simulink model "sim_internal_baseline_TB"  (R2025b)
settings: Solver=FixedStepDiscrete  StartTime=0.0  StopTime=10e-3  RelTol=1e-3
PostLoadFcn:
  | hScopeConfig = get_param([gcs '/Receiver/QPSK Rx/Frequency and Time Synchronizer/Symbol Synchronizer/No HDL/QPSK Receiver Eye Diagram'],'ScopeConfiguration');
  | 
  | hScopeConfig.OpenAtSimulationStart = false;
  | hScopeConfig.Visible = false;
  | SamplesPerSymbol = 4;
  | %UpsamplesRx = 1;
  | clear hScopeConfig
InitFcn:
  | commhdlQPSKTxRxModelInit;
  | % Rate bridge: ADRV9002/Jupiter radio runs at 15.36 MHz = 2x the 7.68 MHz
  | % (4 samples/symbol @ Rsym=1.92 MHz) the QPSK Rx requires. The deployed
  | % Receiver must downsample the ADC stream by 2. UpsamplesRx=1 fed the QPSK
  | % Rx 8 sps (2x-upsampled) and broke symbol sync / the loopback bit check.
  | UpsamplesRx = 2;
  | UpsamplesTx = 1;
  | clear simTimingOffset;
StopFcn:
  | if exist('simTimingOffset','var')
  |   disp('Simulation completed');
  |   %QPSKTxRxVerification;
  | end
values from neighbouring files (symbols this model uses):
  Rsym = variant{2}    [BandwidthVariantSimTest.m]    (also in CoarseFreqEstimatorTest.m = CoarseFreqEstimatorTest.Rsym; PreambleDetectorTest.m = 1920000)
undefined symbols (not defined in the file or in its folder): Add, Config, fsym, randsrc, RandStream, Shift
libraries: hdlsllib x149, simulink x40, dspsigops x36, dsphdlfiltering2 x6, dsphdlsigops2 x4, dsphdlmathfun2 x4, commdigbbndpm3 x4, commchan3 x1, commrflib2 x1
(part 2 of 6)

== system sim_internal_baseline_TB/Receiver/QPSK Rx/Frequency and Time Synchronizer ==
  dataIn : Inport
  validIn : Inport  Port=2
  rstCS : Inport  Port=3
  Carrier Synchronizer : Subsystem
      settings: PortSchema="{\"entries\":[{\"content\":{\"sides\":[{\"content\":{\"connectorIds\":[\"In1\",\"In2\",\"In3\"]},\"type\":\"ConnectorPlacement.EquallySpacedRectSide\",\"uuid\":\"ee58e5dc-083a-48cb-b7f3-66ed8a15890f\"},{\"content\":{\"connectorIds\":[\"Out1\",\"Out2\"],\"side\":\"RIGHT\"},\"type\":\"ConnectorPlacement.EquallySpacedRectSide\",\"uuid\":\"6d121164-5065-4840-a82e-fa57a8e9650e\"},{\"content\":{\"connectorIds\":[\"In4\"],\"side\":\"TOP\"},\"type\":\"ConnectorPlacement.EquallySpacedRectSide\",\"uuid\":\"54d2b8e3-f516-4572-94a0-c914196ae8e4\"}]},\"type\":\"ConnectorPlacement.EquallySpacedConnector\",\"uuid\":\"0f2a6472-efd0-42ca-a030-ab436081b5e1\"}],\"packageUris\":[\"http://schema.mathworks.com/mf0/Connector/R2020b\"],\"version\":\"1.0\"}"
  Coarse Frequency Compensator : Subsystem
      settings: PortSchema="{\"entries\":[{\"content\":{\"sides\":[{\"content\":{\"connectorIds\":[\"In1\",\"In2\"]},\"type\":\"ConnectorPlacement.EquallySpacedRectSide\",\"uuid\":\"138aa5bd-62db-47d6-b55f-f529a6004434\"},{\"content\":{\"connectorIds\":[\"Out1\",\"Out2\",\"Out3\"],\"side\":\"RIGHT\"},\"type\":\"ConnectorPlacement.EquallySpacedRectSide\",\"uuid\":\"8e6ccec0-f736-48ab-be6d-feac886e083d\"},{\"content\":{\"connectorIds\":[\"Out4\"],\"side\":\"TOP\"},\"type\":\"ConnectorPlacement.EquallySpacedRectSide\",\"uuid\":\"d4535392-74fa-432a-a39c-b98ba26e8163\"},{\"content\":{\"side\":\"BOTTOM\"},\"type\":\"ConnectorPlacement.EquallySpacedRectSide\",\"uuid\":\"770ac6a2-7a02-4a77-858b-592982deaf6e\"}]},\"type\":\"ConnectorPlacement.EquallySpacedConnector\",\"uuid\":\"a9b944be-f88b-4ab6-a5e1-6824362eb9ca\"}],\"packageUris\":[\"http://schema.mathworks.com/mf0/Connector/R2020b\"],\"version\":\"1.0\"}"
  No HDL : Subsystem
      settings: PortSchema="{\"entries\":[{\"content\":{\"sides\":[{\"content\":{\"connectorIds\":[\"In1\",\"In2\"]},\"type\":\"ConnectorPlacement.EquallySpacedRectSide\",\"uuid\":\"df96a46d-149f-4580-adf6-e5cf26cffa9b\"},{\"content\":{\"connectorIds\":[\"In3\",\"In4\"],\"side\":\"RIGHT\"},\"type\":\"ConnectorPlacement.EquallySpacedRectSide\",\"uuid\":\"1c46d09c-cb37-4618-ac4e-e5ef50df41fb\"},{\"content\":{\"connectorIds\":[],\"side\":\"TOP\"},\"type\":\"ConnectorPlacement.EquallySpacedRectSide\",\"uuid\":\"7fe62300-46d7-4234-a31d-eecffed4f6e6\"},{\"content\":{\"connectorIds\":[],\"side\":\"BOTTOM\"},\"type\":\"ConnectorPlacement.EquallySpacedRectSide\",\"uuid\":\"05ecd563-28f5-4cfd-b718-5032a7458763\"}]},\"type\":\"ConnectorPlacement.EquallySpacedConnector\",\"uuid\":\"4b3d5859-a469-4389-9e5d-e5f07416a9a1\"}],\"packageUris\":[\"http://schema.mathworks.com/mf0/Connector/R2020b\"],\"version\":\"1.0\"}"
  Packet Controller : Subsystem
  Phase Ambiguity Estimation and Correction : Subsystem
  Preamble Detector : Subsystem
  Symbol Synchronizer : Subsystem
  dataOut : Outport
  startOut : Outport  Port=2
  endOut : Outport  Port=3
  validOut : Outport  Port=4
  postSymbolSync : Outport  Port=5
  postCarrierSync : Outport  Port=6
  nSynced : Outport  Port=7
  normCoarseFreqEst : Outport  Port=8
  wires:
  Coarse Frequency Compensator/3(validOut) -> Carrier Synchronizer/3(validIn)
  Coarse Frequency Compensator/1(dataOut) -> Carrier Synchronizer/1(dataIn)
  Phase Ambiguity Estimation and Correction/1(dataOut) -> Packet Controller/1(dataIn)
  Phase Ambiguity Estimation and Correction/3(validOut) -> Packet Controller/3(validIn)
  Symbol Synchronizer/2(validOut) -> No HDL/2(In2), Coarse Frequency Compensator/2(validIn)
  Symbol Synchronizer/1(dataOut) -> postSymbolSync/1, No HDL/1(In1), Coarse Frequency Compensator/1(dataIn)
  Phase Ambiguity Estimation and Correction/2(syncPulseOut) -> Packet Controller/2(syncPulse)
  Preamble Detector/3(validOut) -> Phase Ambiguity Estimation and Correction/3(validIn)
  Preamble Detector/1(dataOut) -> Phase Ambiguity Estimation and Correction/1(dataIn)
  validIn/1 -> Symbol Synchronizer/2(validIn)
  dataIn/1 -> Symbol Synchronizer/1(dataIn)
  Coarse Frequency Compensator/2(rstCS) -> Carrier Synchronizer/2(internalRst)
  Packet Controller/1(dataOut) -> dataOut/1
  Packet Controller/2(startOut) -> startOut/1
  Packet Controller/3(endOut) -> endOut/1
  Packet Controller/4(validOut) -> validOut/1
  Preamble Detector/2(syncPulse) -> nSynced/1, Phase Ambiguity Estimation and Correction/2(syncPulseIn)
  Carrier Synchronizer/1(dataOut) -> postCarrierSync/1, No HDL/3(In3), Preamble Detector/1(dataIn)
  Carrier Synchronizer/2(validOut) -> No HDL/4(In4), Preamble Detector/2(validIn)
  Coarse Frequency Compensator/4(normalizedFreqEst) -> normCoarseFreqEst/1
  rstCS/1 -> Carrier Synchronizer/4(manualRst)

== system sim_internal_baseline_TB/Receiver/QPSK Rx/HDL Data Descrambler ==
  note: HDL Data Scrambler
      | Polynomial: x^7+x^4+1
      | Initial state: [1 0 1 1 1 0 1]
  dataIn : Inport
  startIn : Inport  Port=2
  endIn : Inport  Port=3
  validIn : Inport  Port=4
  BIT_XOR : Logic  Operator=XOR  IconShape=distinctive  AllPortsSameDT=off  OutDataTypeStr=boolean
  BIT_XOR2 : Logic  Operator=XOR  IconShape=distinctive  AllPortsSameDT=off  OutDataTypeStr=boolean
  Delay{,1..7} (8 alike) : Delay  DelayLength=1
  EnableScrambling : Constant  Value=true  SampleTime=-1
  Logical Operator : Logic  IconShape=distinctive  AllPortsSameDT=off  OutDataTypeStr=boolean
  Switch : Switch  Criteria=u2 > Threshold  SaturateOnIntegerOverflow=off  InputSameDT=off
  Unit Delay Enabled Resettable Synchronous{,2..3,5,7} (5 alike) : hdlsllib/Discrete/Unit Delay Enabled Resettable Synchronous  InitialCondition=1  SampleTime=-1
  Unit Delay Enabled Resettable Synchronous1 : hdlsllib/Discrete/Unit Delay Enabled Resettable Synchronous  InitialCondition=0  SampleTime=-1
  Unit Delay Enabled Resettable Synchronous4 : hdlsllib/Discrete/Unit Delay Enabled Resettable Synchronous  InitialCondition=0  SampleTime=-1
  Unit Delay Enabled Resettable Synchronous6 : hdlsllib/Discrete/Unit Delay Enabled Resettable Synchronous  InitialCondition=0.0  SampleTime=-1
  dataOut : Outport  InitialOutput=0
  startOut : Outport  Port=2  InitialOutput=0
  endOut : Outport  Port=3  InitialOutput=0
  validOut : Outport  Port=4  InitialOutput=0
  wires:
  Delay4/1 -> validOut/1
  Delay3/1 -> dataOut/1
  endIn/1 -> Delay2/1, Unit Delay Enabled Resettable Synchronous4/3
  Logical Operator/1 -> BIT_XOR2/2
  Unit Delay Enabled Resettable Synchronous4/1 -> Logical Operator/1
  Delay1/1 -> Unit Delay Enabled Resettable Synchronous6/2, Unit Delay Enabled Resettable Synchronous2/2, Unit Delay Enabled Resettable Synchronous1/2, Unit Delay Enabled Resettable Synchronous/2, Delay4/1, Unit Delay Enabled Resettable Synchronous3/2, Unit Delay Enabled Resettable Synchronous5/2, Unit Delay Enabled Resettable Synchronous7/2
  Delay/1 -> Switch/3, BIT_XOR2/1
  startIn/1 -> Delay5/1, Unit Delay Enabled Resettable Synchronous4/1, Unit Delay Enabled Resettable Synchronous4/2, Unit Delay Enabled Resettable Synchronous6/3, Unit Delay Enabled Resettable Synchronous5/3, Unit Delay Enabled Resettable Synchronous1/3, Unit Delay Enabled Resettable Synchronous/3, Unit Delay Enabled Resettable Synchronous2/3, Unit Delay Enabled Resettable Synchronous3/3, Unit Delay Enabled Resettable Synchronous7/3
  dataIn/1 -> Delay/1
  validIn/1 -> Delay1/1
  BIT_XOR/1 -> Unit Delay Enabled Resettable Synchronous/1, Logical Operator/2
  Unit Delay Enabled Resettable Synchronous1/1 -> Unit Delay Enabled Resettable Synchronous2/1
  Unit Delay Enabled Resettable Synchronous2/1 -> Unit Delay Enabled Resettable Synchronous3/1
  Unit Delay Enabled Resettable Synchronous/1 -> Unit Delay Enabled Resettable Synchronous1/1
  Unit Delay Enabled Resettable Synchronous3/1 -> BIT_XOR/2, Unit Delay Enabled Resettable Synchronous5/1
  Unit Delay Enabled Resettable Synchronous5/1 -> Unit Delay Enabled Resettable Synchronous6/1
  Unit Delay Enabled Resettable Synchronous6/1 -> Unit Delay Enabled Resettable Synchronous7/1
  Unit Delay Enabled Resettable Synchronous7/1 -> BIT_XOR/1
  Delay2/1 -> Delay6/1
  Delay5/1 -> Delay7/1
  Delay6/1 -> endOut/1
  Delay7/1 -> startOut/1
  EnableScrambling/1 -> Switch/2
  BIT_XOR2/1 -> Switch/1
  Switch/1 -> Delay3/1

== system sim_internal_baseline_TB/Receiver/QPSK Rx/QPSK Demodulator ==
  dataIn : Inport
  startIn : Inport  Port=2
  endIn : Inport  Port=3
  validIn : Inport  Port=4
  Delay{,1..13} (14 alike) : Delay  DelayLength=1
  QPSK Demodulator Baseband : commdigbbndpm3/QPSK Demodulator Baseband  OutType=Bit  DecType=Hard decision  VarSource=Dialog  Variance=1  Dec=Gray  Ph=pi/4  outDtype1=boolean  outDtype2=Inherit via internal rule  derotateFactorWordLen=16  derotateFactorDataTypeStr=Inherit: Same word length as input  derotateFactorLastDataTypeStr=Inherit: Same word length as input
  Serializer : Subsystem
  Signal Specification : SignalSpecification  Dimensions=1
  dataOut : Outport
  startOut : Outport  Port=2
  endOut : Outport  Port=3
  validOut : Outport  Port=4
  wires:
  Delay/1 -> QPSK Demodulator Baseband/1
  Delay1/1 -> Delay5/1
  Delay6/1 -> Delay4/1
  Delay7/1 -> Delay13/1
  Delay2/1 -> Delay6/1
  Delay3/1 -> Delay7/1
  Signal Specification/1 -> Delay/1
  QPSK Demodulator Baseband/1 -> Delay12/1
  Delay8/1 -> dataOut/1
  Delay9/1 -> validOut/1
  Delay10/1 -> startOut/1
  Delay11/1 -> endOut/1
  Delay5/1 -> Serializer/2(In2)
  Delay12/1 -> Serializer/1(u)
  Delay4/1 -> Delay10/1
  Delay13/1 -> Delay11/1
  Serializer/1(Out1) -> Delay8/1
  Serializer/2(Out2) -> Delay9/1
  dataIn/1 -> Signal Specification/1
  validIn/1 -> Delay1/1
  startIn/1 -> Delay2/1
  endIn/1 -> Delay3/1

== system sim_internal_baseline_TB/Transmitter/Input Data/Message Generator ==
  reset : Inport
  enable : Inport  Port=2
  MATLAB Function : MATLAB Function  TreatAsAtomicUnit=on
  out : Outport
  stop : Outport  Port=2
  start : Outport  Port=3
  valid : Outport  Port=4
  count : Outport  Port=5
  msg_count_out : Outport  Port=6
  wires:
  MATLAB Function/3(stop) -> stop/1
  MATLAB Function/1(out) -> out/1
  reset/1 -> MATLAB Function/2(reset)
  MATLAB Function/2(start) -> start/1
  enable/1 -> MATLAB Function/1(enable)
  MATLAB Function/4(valid) -> valid/1
  MATLAB Function/5(count_out) -> count/1
  MATLAB Function/6(msg_count_out) -> msg_count_out/1

== system sim_internal_baseline_TB/Transmitter/QPSK Tx/Bit Packetizer ==
  dataIn : Inport
  validIn : Inport  Port=2
  Compare To Constant : hdlsllib/Logic and Bit Operations/Compare To Constant  relop===  const=length(Preamble)  OutDataTypeStr=boolean
  Compare To Constant1 : hdlsllib/Logic and Bit Operations/Compare To Constant  relop===  const=bitsPerPacket - 1  OutDataTypeStr=boolean
  Compare To Constant2 : hdlsllib/Logic and Bit Operations/Compare To Constant  relop=>=  const=length(Preamble)  OutDataTypeStr=boolean
  Data Bits FIFO : Subsystem
  Data Type Conversion : DataTypeConversion  OutDataTypeStr=boolean  SaturateOnIntegerOverflow=off  RndMeth=Floor
  HDL Counter : hdlsllib/Sources/HDL Counter  CountType=Count limited  CountInit=0  CountStep=1  CountMax=1  CountFromType=Initial value  CountFrom=0  CountResetPort=off  CountLoadPort=off  CountEnbPort=on  CountDirPort=off  CountHitOutputPort=off  CountDataType=Unsigned  CountWordLen=1  CountFracLen=0  CountSampTime=1
  Logical Operator : Logic  AllPortsSameDT=off  OutDataTypeStr=boolean
  Logical Operator1 : Logic  AllPortsSameDT=off  OutDataTypeStr=boolean
  Logical Operator2 : Logic  Operator=NOT  AllPortsSameDT=off  OutDataTypeStr=boolean
  Preamble Bits Generator : Subsystem
  Switch : Switch  Criteria=u2 ~= 0  SaturateOnIntegerOverflow=off  InputSameDT=off
  bitsOut : Outport
  dataStart : Outport  Port=2
  dataEnd : Outport  Port=3
  bitsValid : Outport  Port=4
  dataReady : Outport  Port=5
  wires:
  dataIn/1 -> Data Bits FIFO/1(data)
  validIn/1 -> Data Bits FIFO/2(push)
  Compare To Constant/1 -> Logical Operator/1
  Compare To Constant1/1 -> Logical Operator1/2
  Logical Operator/1 -> dataStart/1
  Logical Operator1/1 -> dataEnd/1
  Data Bits FIFO/5(fullRAM) -> Logical Operator2/1
  Logical Operator2/1 -> HDL Counter/1
  Data Bits FIFO/1(dataOut) -> Switch/1
  Data Bits FIFO/3(sampleCount) -> Preamble Bits Generator/2(sampleCount), Compare To Constant/1, Compare To Constant1/1, Compare To Constant2/1
  Data Bits FIFO/4(sampleCountValid) -> bitsValid/1, Logical Operator/2, Logical Operator1/1, Preamble Bits Generator/3(sampleCountValid)
  Data Bits FIFO/2(activeFrame) -> Preamble Bits Generator/1(activeFrame)
  Preamble Bits Generator/1(preambleBits) -> Switch/3
  Compare To Constant2/1 -> Switch/2
  Switch/1 -> bitsOut/1
  HDL Counter/1 -> Data Type Conversion/1
  Data Type Conversion/1 -> dataReady/1

== system sim_internal_baseline_TB/Transmitter/QPSK Tx/HDL Data Scrambler ==
  note: HDL Data Scrambler
      | Polynomial: x^7+x^4+1
      | Initial state: [1 0 1 1 1 0 1]
  dataIn : Inport
  startIn : Inport  Port=2
  endIn : Inport  Port=3
  validIn : Inport  Port=4
  BIT_XOR : Logic  Operator=XOR  IconShape=distinctive  AllPortsSameDT=off  OutDataTypeStr=boolean
  BIT_XOR2 : Logic  Operator=XOR  IconShape=distinctive  AllPortsSameDT=off  OutDataTypeStr=boolean
  Delay{,1,3..4} (4 alike) : Delay  DelayLength=1
  EnableScrambling : Constant  Value=true  SampleTime=-1
  Logical Operator : Logic  IconShape=distinctive  AllPortsSameDT=off  OutDataTypeStr=boolean
  Switch : Switch  Criteria=u2 > Threshold  SaturateOnIntegerOverflow=off  InputSameDT=off
  Unit Delay Enabled Resettable Synchronous{,2..3,5,7} (5 alike) : hdlsllib/Discrete/Unit Delay Enabled Resettable Synchronous  InitialCondition=1  SampleTime=-1
  Unit Delay Enabled Resettable Synchronous1 : hdlsllib/Discrete/Unit Delay Enabled Resettable Synchronous  InitialCondition=0  SampleTime=-1
  Unit Delay Enabled Resettable Synchronous4 : hdlsllib/Discrete/Unit Delay Enabled Resettable Synchronous  InitialCondition=0  SampleTime=-1
  Unit Delay Enabled Resettable Synchronous6 : hdlsllib/Discrete/Unit Delay Enabled Resettable Synchronous  InitialCondition=0.0  SampleTime=-1
  dataOut : Outport  InitialOutput=0
  validOut : Outport  Port=2  InitialOutput=0
  wires:
  Delay4/1 -> validOut/1
  Delay3/1 -> dataOut/1
  endIn/1 -> Unit Delay Enabled Resettable Synchronous4/3
  Logical Operator/1 -> BIT_XOR2/2
  Unit Delay Enabled Resettable Synchronous4/1 -> Logical Operator/1
  Delay1/1 -> Unit Delay Enabled Resettable Synchronous6/2, Unit Delay Enabled Resettable Synchronous2/2, Unit Delay Enabled Resettable Synchronous1/2, Unit Delay Enabled Resettable Synchronous/2, Delay4/1, Unit Delay Enabled Resettable Synchronous3/2, Unit Delay Enabled Resettable Synchronous5/2, Unit Delay Enabled Resettable Synchronous7/2
  Delay/1 -> Switch/3, BIT_XOR2/1
  startIn/1 -> Unit Delay Enabled Resettable Synchronous4/1, Unit Delay Enabled Resettable Synchronous4/2, Unit Delay Enabled Resettable Synchronous6/3, Unit Delay Enabled Resettable Synchronous5/3, Unit Delay Enabled Resettable Synchronous1/3, Unit Delay Enabled Resettable Synchronous/3, Unit Delay Enabled Resettable Synchronous2/3, Unit Delay Enabled Resettable Synchronous3/3, Unit Delay Enabled Resettable Synchronous7/3
  dataIn/1 -> Delay/1
  validIn/1 -> Delay1/1
  BIT_XOR/1 -> Unit Delay Enabled Resettable Synchronous/1, Logical Operator/2
  Unit Delay Enabled Resettable Synchronous1/1 -> Unit Delay Enabled Resettable Synchronous2/1
  Unit Delay Enabled Resettable Synchronous2/1 -> Unit Delay Enabled Resettable Synchronous3/1
  Unit Delay Enabled Resettable Synchronous/1 -> Unit Delay Enabled Resettable Synchronous1/1
  Unit Delay Enabled Resettable Synchronous3/1 -> BIT_XOR/2, Unit Delay Enabled Resettable Synchronous5/1
  Unit Delay Enabled Resettable Synchronous5/1 -> Unit Delay Enabled Resettable Synchronous6/1
  Unit Delay Enabled Resettable Synchronous6/1 -> Unit Delay Enabled Resettable Synchronous7/1
  Unit Delay Enabled Resettable Synchronous7/1 -> BIT_XOR/1
  Switch/1 -> Delay3/1
  EnableScrambling/1 -> Switch/2
  BIT_XOR2/1 -> Switch/1

== system sim_internal_baseline_TB/Transmitter/QPSK Tx/QPSK Modulator ==
  dataIn : Inport
  validIn : Inport  Port=2
  Compare To Constant : simulink/Logic and Bit Operations/Compare To Constant  relop===  const=0  OutDataTypeStr=boolean
  Compare To Constant1 : simulink/Logic and Bit Operations/Compare To Constant  relop===  const=1  OutDataTypeStr=boolean
  Delay{,1..5,11..12} (8 alike) : Delay  DelayLength=1
  HDL Counter : hdlsllib/Sources/HDL Counter  CountType=Count limited  CountInit=0  CountStep=1  CountMax=1  CountFromType=Initial value  CountFrom=0  CountResetPort=off  CountLoadPort=off  CountEnbPort=on  CountDirPort=off  CountHitOutputPort=off  CountDataType=Unsigned  CountWordLen=1  CountFracLen=0  CountSampTime=1
  Logical Operator : Logic  IconShape=distinctive  AllPortsSameDT=off  OutDataTypeStr=boolean
  Logical Operator1 : Logic  IconShape=distinctive  AllPortsSameDT=off  OutDataTypeStr=boolean
  Mux : Mux  Inputs=2
  Null : Constant  Value=complex(0,0)  OutDataTypeStr=fixdt(1,16,15)  SampleTime=1/(Rsym*4)
  QPSK Modulator Baseband : commdigbbndpm3/QPSK Modulator Baseband  InType=Bit  Enc=Gray  Ph=pi/4  outDtype=Fixed-point  outWordLen=16  outUDDataType=sfix(16)  outFracLenMode=User-defined  outFracLen=15  outDataTypeStr=fixdt(1,16,15)  outLastDataTypeStr=fixdt(1,16,15)
  Switch3 : Switch  Threshold=1  SaturateOnIntegerOverflow=off  InputSameDT=off
  Unit Delay Enabled Synchronous : hdlsllib/Discrete/Unit Delay Enabled Synchronous  InitialCondition=0.0  SampleTime=-1
  dataOut : Outport
  validOut : Outport  Port=2
  wires:
  dataIn/1 -> Delay/1
  validIn/1 -> Delay1/1
  HDL Counter/1 -> Compare To Constant/1, Compare To Constant1/1
  QPSK Modulator Baseband/1 -> Delay11/1
  Logical Operator1/1 -> Delay5/1
  Switch3/1 -> Delay2/1
  Null/1 -> Switch3/3
  Delay/1 -> Mux/2, Unit Delay Enabled Synchronous/1
  Delay2/1 -> dataOut/1
  Delay3/1 -> validOut/1
  Delay1/1 -> Logical Operator1/2, Logical Operator/1, HDL Counter/1
  Compare To Constant/1 -> Logical Operator/2
  Compare To Constant1/1 -> Logical Operator1/1
  Delay11/1 -> Switch3/1
  Delay12/1 -> Switch3/2, Delay3/1
  Logical Operator/1 -> Unit Delay Enabled Synchronous/2
  Unit Delay Enabled Synchronous/1 -> Mux/1
  Mux/1 -> Delay4/1
  Delay4/1 -> QPSK Modulator Baseband/1
  Delay5/1 -> Delay12/1

== system sim_internal_baseline_TB/Transmitter/QPSK Tx/RRC Transmit Filter ==
  dataIn : Inport
  validIn : Inport  Port=2
  Data Type Conversion : DataTypeConversion  OutDataTypeStr=fixdt(1,17,16)  SaturateOnIntegerOverflow=off  RndMeth=Floor
  Data Type Conversion1 : DataTypeConversion  OutDataTypeStr=fixdt(1,16,14)  SaturateOnIntegerOverflow=off  RndMeth=Floor
  Delay1 : Delay  DelayLength=1
  Delay2 : Delay  DelayLength=1
  Delay3 : Delay  DelayLength=1
  RRC Filter : dsphdlfiltering2/Discrete FIR Filter  NumeratorSource=Property  Numerator=RRCCoef  NumeratorPrototype=[]  FilterStructure=Direct form systolic  SerializationOption=Minimum number of cycles between valid input samples  NumCycles=2  NumberOfMultipliers=2  SimulateUsing=Code generation  roundingMode=Floor  overflowMode=off  CoefficientsDataTypeStr=Inherit: Same word length as input  OutputDataTypeStr=Inherit: Same word length as input  ResetInputPort=off  HDLGlobalReset=off  CoeffMultiplier=Multiplier  UseMultForPow2Coeff=on  FrameInputSymmOptim=off
  Unit Delay Enabled Synchronous1 : hdlsllib/Discrete/Unit Delay Enabled Synchronous  InitialCondition=0  SampleTime=-1
  dataOut : Outport
  validOut : Outport  Port=2
  wires:
  dataIn/1 -> Data Type Conversion/1
  RRC Filter/1 -> Data Type Conversion1/1
  RRC Filter/2 -> Delay2/1
  Delay1/1 -> dataOut/1
  Delay2/1 -> validOut/1
  Data Type Conversion/1 -> Delay3/1
  Unit Delay Enabled Synchronous1/1 -> RRC Filter/2
  Data Type Conversion1/1 -> Delay1/1
  validIn/1 -> Unit Delay Enabled Synchronous1/2, Unit Delay Enabled Synchronous1/1
  Delay3/1 -> RRC Filter/1

== system sim_internal_baseline_TB/TxRxComposite/Receiver/Capture Data Bits ==
  dataOut : Inport
  dataSrt : Inport  Port=2
  dataEnd : Inport  Port=3
  valid : Inport  Port=4
  Display : Display
  Display1 : Display
  Display2 : Display
  MATLAB Function : MATLAB Function  TreatAsAtomicUnit=on
  count_out : Outport
  packets_out : Outport  Port=2
  bit_errors_out : Outport  Port=3
  wires:
  MATLAB Function/3(bit_errors_out) -> Display2/1, bit_errors_out/1
  MATLAB Function/2(packets_out) -> Display1/1, packets_out/1
  MATLAB Function/1(count_out) -> Display/1, count_out/1
  valid/1 -> MATLAB Function/1(valid)
  dataEnd/1 -> MATLAB Function/4(stop)
  dataSrt/1 -> MATLAB Function/3(start)
  dataOut/1 -> MATLAB Function/2(datain)

== system sim_internal_baseline_TB/TxRxComposite/Receiver/QPSK Rx ==
  dataIn : Inport  OutDataTypeStr=fixdt(1,16,14)  PortDimensions=1  SampleTime=1/(Rsym*SamplesPerSymbol)
      settings: SignalType=complex
  validIn : Inport  Port=2  OutDataTypeStr=boolean  PortDimensions=1  SampleTime=1/(Rsym*SamplesPerSymbol)
  rstCS : Inport  Port=3  OutDataTypeStr=boolean  PortDimensions=1
      settings: SignalType=complex
  debugMuxCtrl : Inport  Port=4  OutDataTypeStr=uint32  PortDimensions=1  SampleTime=1/(Rsym*SamplesPerSymbol)
  Automatic Gain Control : Subsystem  mask{Ref=AGCReference, LFG=AGCLoopGain}
      mask prompts: Ref "Error Detector Reference:"; LFG "Loop Filter Gain"
  Bus Creator : BusCreator  Inputs=4
  Bus Creator1 : BusCreator  Inputs=3
  Complex to Real-Imag : ComplexToRealImag
  Constant : Constant  Value=true  SampleTime=1/(Rsym*4)
  Data Type Conversion : DataTypeConversion  OutDataTypeStr=int16  ConvertRealWorld=Stored Integer (SI)  SaturateOnIntegerOverflow=off  RndMeth=Floor
  Delay{,1..8} (9 alike) : Delay  DelayLength=1
  Frequency and Time Synchronizer : Subsystem
      settings: PortSchema="{\"entries\":[{\"content\":{\"sides\":[{\"content\":{\"connectorIds\":[\"In1\",\"In2\"]},\"type\":\"ConnectorPlacement.EquallySpacedRectSide\",\"uuid\":\"8bc6a452-5111-4806-8ca9-335cb622aea6\"},{\"content\":{\"connectorIds\":[\"Out1\",\"Out2\",\"Out3\",\"Out4\"],\"side\":\"RIGHT\"},\"type\":\"ConnectorPlacement.EquallySpacedRectSide\",\"uuid\":\"b0f43c98-f5c0-4f62-94ae-d69789942eef\"},{\"content\":{\"connectorIds\":[\"In3\",\"Out7\",\"Out8\"],\"side\":\"TOP\"},\"type\":\"ConnectorPlacement.EquallySpacedRectSide\",\"uuid\":\"427ff3b3-b896-4008-9584-d311480df763\"},{\"content\":{\"connectorIds\":[\"Out5\",\"Out6\"],\"side\":\"BOTTOM\"},\"type\":\"ConnectorPlacement.EquallySpacedRectSide\",\"uuid\":\"f704cb90-80a1-4198-8b72-e70182b45e73\"},{\"content\":{\"side\":\"HIDDEN\"},\"type\":\"ConnectorPlacement.EquallySpacedRectSide\",\"uuid\":\"f6309498-1e43-486f-b6b5-2c6570711f8e\"}]},\"type\":\"ConnectorPlacement.EquallySpacedConnector\",\"uuid\":\"f0ce492e-c9e1-4b35-98ef-84d77b696cfe\"}],\"packageUris\":[\"http://schema.mathworks.com/mf0/Connector/R2020b\"],\"version\":\"1.0\"}"
  HDL Data Descrambler : Subsystem
  Index Vector : MultiPortSwitch  DataPortOrder=Zero-based contiguous  Inputs=4  DiagnosticForDefault=None  zeroidx=on  SaturateOnIntegerOverflow=off  InputSameDT=off
  QPSK Demodulator : Subsystem
  RRC Receive Filter : dsphdlfiltering2/Discrete FIR Filter  NumeratorSource=Property  Numerator=RRCCoef  NumeratorPrototype=[]  FilterStructure=Direct form systolic  SerializationOption=Minimum number of cycles between valid input samples  NumCycles=2  NumberOfMultipliers=2  SimulateUsing=Code generation  roundingMode=Floor  overflowMode=off  CoefficientsDataTypeStr=Inherit: Same word length as input  OutputDataTypeStr=Inherit: Same word length as input  ResetInputPort=off  HDLGlobalReset=off  CoeffMultiplier=Multiplier  UseMultForPow2Coeff=on  FrameInputSymmOptim=off
  dataOut : Outport
  ctrlOut : Outport  Port=2
  rxDiagBus : Outport  Port=3
  debugIOut : Outport  Port=4
  debugQOut : Outport  Port=5
  debugValid : Outport  Port=6
  wires:
  Constant/1 -> Delay8/1
  Delay8/1 -> Delay7/1
  Delay7/1 -> debugValid/1
  Delay6/1 -> Complex to Real-Imag/1
  Index Vector/1 -> Delay5/1
  Delay5/1 -> Data Type Conversion/1
  Delay4/1 -> Index Vector/5
  Delay3/1 -> Index Vector/4
  Delay2/1 -> Index Vector/3
  Delay1/1 -> Index Vector/2
  Data Type Conversion/1 -> Delay6/1
  Complex to Real-Imag/1 -> debugIOut/1
  Complex to Real-Imag/2 -> debugQOut/1
  debugMuxCtrl/1 -> Index Vector/1
  Frequency and Time Synchronizer/6(postCarrierSync) -> Delay3/1
  Frequency and Time Synchronizer/5(postSymbolSync) -> Delay2/1
  Delay/1 -> rxDiagBus/1
  QPSK Demodulator/4(validOut) -> HDL Data Descrambler/4(validIn)
  Frequency and Time Synchronizer/4(validOut) -> Bus Creator/4, QPSK Demodulator/4(validIn)  "QPSKConstellationValid"
  Frequency and Time Synchronizer/2(startOut) -> QPSK Demodulator/2(startIn)
  QPSK Demodulator/2(startOut) -> HDL Data Descrambler/2(startIn)
  HDL Data Descrambler/4(validOut) -> Bus Creator1/3  "validOut"
  HDL Data Descrambler/1(dataOut) -> dataOut/1
  dataIn/1 -> Automatic Gain Control/1(dataIn)
  Frequency and Time Synchronizer/1(dataOut) -> Bus Creator/3, QPSK Demodulator/1(dataIn), Delay4/1  "QPSKConstellationPoints"
  Automatic Gain Control/1(dataOut) -> RRC Receive Filter/1, Delay1/1
  Bus Creator/1 -> Delay/1
  Frequency and Time Synchronizer/7(nSynced) -> Bus Creator/1  "nSynced"
  RRC Receive Filter/2 -> Frequency and Time Synchronizer/2(validIn)
  Frequency and Time Synchronizer/3(endOut) -> QPSK Demodulator/3(endIn)
  HDL Data Descrambler/2(startOut) -> Bus Creator1/1  "startOut"
  Bus Creator1/1 -> ctrlOut/1
  Frequency and Time Synchronizer/8(normCoarseFreqEst) -> Bus Creator/2  "normCoarseFreqEst"
  QPSK Demodulator/3(endOut) -> HDL Data Descrambler/3(endIn)
  HDL Data Descrambler/3(endOut) -> Bus Creator1/2  "endOut"
  RRC Receive Filter/1 -> Frequency and Time Synchronizer/1(dataIn)
  Automatic Gain Control/2(validOut) -> RRC Receive Filter/2
  validIn/1 -> Automatic Gain Control/2(validIn)
  QPSK Demodulator/1(dataOut) -> HDL Data Descrambler/1(dataIn)
  rstCS/1 -> Frequency and Time Synchronizer/3(rstCS)

== system sim_internal_baseline_TB/TxRxComposite/Transmitter/Input Data ==
  enb : Inport
  reset : Inport  Port=2
  Cast To Boolean : DataTypeConversion  OutDataTypeStr=boolean  SaturateOnIntegerOverflow=off  RndMeth=Floor
  Delay : Delay  DelayLength=1
  Display : Display
  Message Generator : Subsystem
  Terminator : Terminator
  Terminator1 : Terminator
  txData : Outport
  txValid : Outport  Port=2
  msg_count_out : Outport  Port=3
  wires:
  Message Generator/6(msg_count_out) -> msg_count_out/1
  Message Generator/3(start) -> Terminator1/1
  reset/1 -> Terminator/1
  Cast To Boolean/1 -> Message Generator/1(reset)
  Delay/1 -> Cast To Boolean/1
  Message Generator/2(stop) -> Delay/1
  Message Generator/5(count) -> Display/1
  enb/1 -> Message Generator/2(enable)
  Message Generator/1(out) -> txData/1
  Message Generator/4(valid) -> txValid/1

== system sim_internal_baseline_TB/TxRxComposite/Transmitter/QPSK Tx ==
  dataIn : Inport  OutDataTypeStr=boolean  PortDimensions=1
  validIn : Inport  Port=2  OutDataTypeStr=boolean  PortDimensions=1
  Bit Packetizer : Subsystem
  Bus Creator : BusCreator  Inputs=2
  HDL Data Scrambler : Subsystem
  QPSK Modulator : Subsystem
  RRC Transmit Filter : Subsystem
  dataReady : Outport
  dataOut : Outport  Port=2
  txDiagBus : Outport  Port=3
  validOut : Outport  Port=4
  wires:
  Bit Packetizer/4(bitsValid) -> HDL Data Scrambler/4(validIn)
  Bus Creator/1 -> txDiagBus/1
  Bit Packetizer/5(dataReady) -> dataReady/1
  Bit Packetizer/2(dataStart) -> HDL Data Scrambler/2(startIn)
  QPSK Modulator/1(dataOut) -> RRC Transmit Filter/1(dataIn), Bus Creator/1  "QPSKConstellationPoints"
  RRC Transmit Filter/1(dataOut) -> dataOut/1
  HDL Data Scrambler/2(validOut) -> QPSK Modulator/2(validIn)
  Bit Packetizer/3(dataEnd) -> HDL Data Scrambler/3(endIn)
  dataIn/1 -> Bit Packetizer/1(dataIn)
  QPSK Modulator/2(validOut) -> RRC Transmit Filter/2(validIn), Bus Creator/2  "QPSKConstellationValid"
  Bit Packetizer/1(bitsOut) -> HDL Data Scrambler/1(dataIn)
  HDL Data Scrambler/1(dataOut) -> QPSK Modulator/1(dataIn)
  RRC Transmit Filter/2(validOut) -> validOut/1
  validIn/1 -> Bit Packetizer/2(validIn)

== system sim_internal_baseline_TB/Receiver/QPSK Rx/Automatic Gain Control/Error Detector ==
  dataIn : Inport
  Add1 : Sum  Inputs=+-
  Conj : Math  Operator=conj
  Data Type Duplicate : DataTypeDuplicate
  Delay{,1..3} (4 alike) : Delay
  Product : Product
  Ref : Constant  Value=Ref  OutDataTypeStr=Inherit: Inherit via back propagation  SampleTime=-1
  err : Outport
  wires:
  Delay3/1 -> err/1
  Delay2/1 -> Add1/2
  Delay1/1 -> Product/1
  Delay/1 -> Product/2
  Ref/1 -> Data Type Duplicate/1, Add1/1
  Conj/1 -> Delay/1
  Product/1 -> Delay2/1
  dataIn/1 -> Conj/1, Data Type Duplicate/2, Delay1/1
  Add1/1 -> Delay3/1

== system sim_internal_baseline_TB/Receiver/QPSK Rx/Automatic Gain Control/Loop Filter ==
  note: Fixed point precision loss warnings
      | are supressed in Mask Init Callback
  err : Inport
  Add : Sum  Inputs=|++  OutDataTypeStr=Inherit: Same as first input
  Delay1 : Delay  DelayLength=1
  Delay2 : Delay
  Delay3 : Delay
  Gain1 : Gain  Gain=LFG  OutDataTypeStr=Inherit: Same as input
      mask init:
      | Simulink.suppressDiagnostic(gcb, 'SimulinkFixedPoint:util:fxpParameterPrecisionLoss');
  gain : Outport
  wires:
  Delay3/1 -> Gain1/1
  Delay2/1 -> Add/1
  Gain1/1 -> Delay2/1
  Add/1 -> Delay1/1
  Delay1/1 -> Add/2, gain/1
  err/1 -> Delay3/1

== system sim_internal_baseline_TB/Receiver/QPSK Rx/Frequency and Time Synchronizer/Carrier Synchronizer ==
  dataIn : Inport
  internalRst : Inport  Port=2
  validIn : Inport  Port=3
  manualRst : Inport  Port=4
  Data Type Conversion2 : DataTypeConversion  OutDataTypeStr=fixdt(1,16,14)  SaturateOnIntegerOverflow=off  RndMeth=Floor
  Delay{,2,5,7,11} (5 alike) : Delay  DelayLength=1
  Delay{1,10,14..15} (4 alike) : Delay  DelayLength=6
  Delay{3..4,6,8..9,12..13} (7 alike) : Delay
  Direct Digital Synthesis : Subsystem
  Logical Operator : Logic  AllPortsSameDT=off  OutDataTypeStr=boolean
  Loop Filter : Subsystem
  Math Function : Math  Operator=conj  SignedPower=on  RndMeth=Zero
  Phase Error Detector : Subsystem
  Product : Product
  dataOut : Outport
  validOut : Outport  Port=2
  wires:
  Delay/1 -> Phase Error Detector/1(dataIn)
  Math Function/1 -> Delay3/1
  Data Type Conversion2/1 -> Delay5/1, Delay/1
  Delay3/1 -> Product/2
  Product/1 -> Delay6/1
  Delay8/1 -> Delay2/1, Delay7/1
  Delay9/1 -> Delay8/1
  Delay4/1 -> Product/1
  Delay6/1 -> Data Type Conversion2/1
  Direct Digital Synthesis/1(expOut) -> Math Function/1
  Loop Filter/1(v) -> Direct Digital Synthesis/3(phaseInc)
  Phase Error Detector/1(PhaseError) -> Loop Filter/1(e)
  Delay2/1 -> Delay1/1
  Delay1/1 -> Loop Filter/2(validIn)
  Delay10/1 -> Delay4/1
  Delay11/1 -> Delay15/1
  Delay12/1 -> Delay11/1
  Delay13/1 -> Delay12/1
  Loop Filter/2(valid) -> Direct Digital Synthesis/2(validIn)
  Delay5/1 -> dataOut/1
  Delay7/1 -> validOut/1
  dataIn/1 -> Delay10/1
  internalRst/1 -> Delay13/1
  validIn/1 -> Delay14/1
  Delay14/1 -> Delay9/1
  manualRst/1 -> Logical Operator/1, Loop Filter/4(externalRst)
  Delay15/1 -> Loop Filter/3(internalRst)
  Loop Filter/3(rst) -> Logical Operator/2
  Logical Operator/1 -> Direct Digital Synthesis/1(rst)

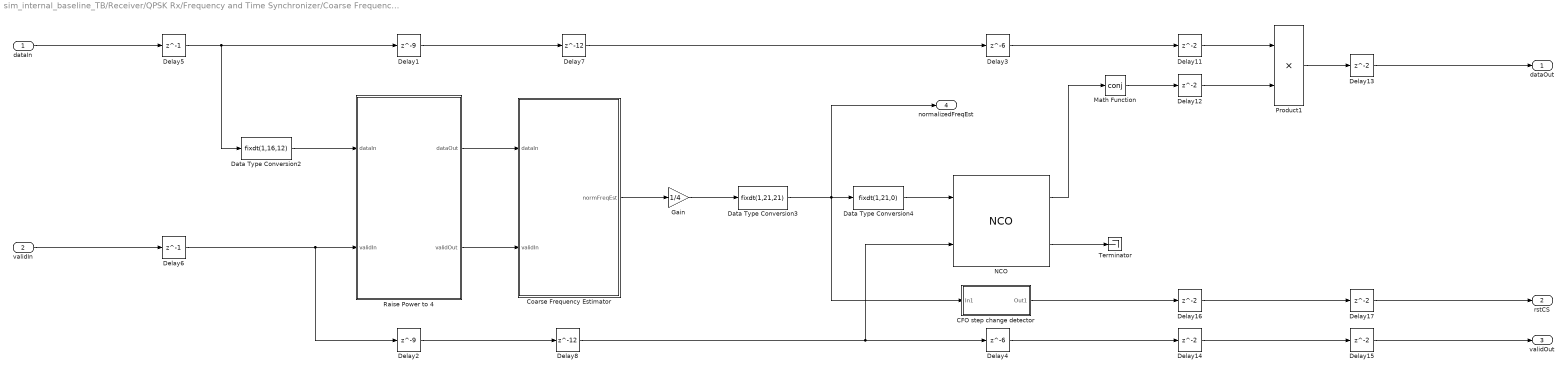
== system sim_internal_baseline_TB/Receiver/QPSK Rx/Frequency and Time Synchronizer/Coarse Frequency Compensator ==
  dataIn : Inport
  validIn : Inport  Port=2
  CFO step change detector : Subsystem
  Coarse Frequency Estimator : Subsystem
  Data Type Conversion2 : DataTypeConversion  OutDataTypeStr=fixdt(1,16,12)  SaturateOnIntegerOverflow=off  RndMeth=Floor
  Data Type Conversion3 : DataTypeConversion  OutDataTypeStr=fixdt(1,21,21)  SaturateOnIntegerOverflow=off  RndMeth=Floor
  Data Type Conversion4 : DataTypeConversion  OutDataTypeStr=fixdt(1,21,0)  ConvertRealWorld=Stored Integer (SI)  SaturateOnIntegerOverflow=off  RndMeth=Floor
  Delay1 : Delay  DelayLength=9
  Delay{11..17} (7 alike) : Delay
  Delay2 : Delay  DelayLength=9
  Delay3 : Delay  DelayLength=6
  Delay4 : Delay  DelayLength=6
  Delay5 : Delay  DelayLength=1
  Delay6 : Delay  DelayLength=1
  Delay7 : Delay  DelayLength=12
  Delay8 : Delay  DelayLength=12
  Gain : Gain  Gain=1/4  ParamDataTypeStr=fixdt(0,2,2)  OutDataTypeStr=Inherit: Same as input
  Math Function : Math  Operator=conj
  NCO : dsphdlsigops2/NCO  PhaseIncrementSource=Input port  PhaseIncrement=100  PhaseOffsetSource=Property  PhaseOffset=0  DitherSource=None  NumDitherBits=4  SamplesPerFrame=1  LUTCompress=off  ResetAction=off  Waveform=Complex exponential  PhasePort=off  SimulateUsing=Code generation  AccumulatorWL=21  PhaseQuantization=on  NumQuantizerAccumulatorBits=14  OutputDataType=Binary point scaling  OutputWL=16  OutputFL=14
  Product1 : Product  OutDataTypeStr=Inherit: Same as first input
  Raise Power to 4 : Subsystem
  Terminator : Terminator
  dataOut : Outport
  rstCS : Outport  Port=2
  validOut : Outport  Port=3
  normalizedFreqEst : Outport  Port=4
  wires:
  Delay14/1 -> Delay15/1
  Delay11/1 -> Product1/1
  Delay6/1 -> Raise Power to 4/2(validIn), Delay2/1
  Delay5/1 -> Delay1/1, Data Type Conversion2/1
  Data Type Conversion4/1 -> NCO/1
  Delay4/1 -> Delay14/1
  Delay3/1 -> Delay11/1
  Delay2/1 -> Delay8/1
  Delay1/1 -> Delay7/1
  NCO/2 -> Terminator/1
  NCO/1 -> Math Function/1
  Product1/1 -> Delay13/1
  Raise Power to 4/2(validOut) -> Coarse Frequency Estimator/2(validIn)
  Math Function/1 -> Delay12/1
  Raise Power to 4/1(dataOut) -> Coarse Frequency Estimator/1(dataIn)
  Delay12/1 -> Product1/2
  Coarse Frequency Estimator/1(normFreqEst) -> Gain/1
  Data Type Conversion2/1 -> Raise Power to 4/1(dataIn)
  Delay16/1 -> Delay17/1
  CFO step change detector/1(Out1) -> Delay16/1
  Gain/1 -> Data Type Conversion3/1
  Delay13/1 -> dataOut/1
  dataIn/1 -> Delay5/1
  validIn/1 -> Delay6/1
  Delay17/1 -> rstCS/1
  Data Type Conversion3/1 -> normalizedFreqEst/1, CFO step change detector/1(In1), Data Type Conversion4/1
  Delay15/1 -> validOut/1
  Delay7/1 -> Delay3/1
  Delay8/1 -> NCO/2, Delay4/1

== system sim_internal_baseline_TB/Receiver/QPSK Rx/Frequency and Time Synchronizer/No HDL ==
  In1 : Inport
  In2 : Inport  Port=2
  In3 : Inport  Port=3
  In4 : Inport  Port=4
  Data Type Conversion : DataTypeConversion  OutDataTypeStr=double  SaturateOnIntegerOverflow=off  RndMeth=Floor
  Data Type Conversion1 : DataTypeConversion  OutDataTypeStr=double  SaturateOnIntegerOverflow=off  RndMeth=Floor
  QPSK Receiver Constellations 2 : ConstellationDiagram  NumInputPorts=2  WindowPosition=[67.000000,180.000000,973.000000,678.000000,]  Visible=on  ScopeFrameLocation=window  SymbolsToDisplaySource=Property  SymbolsToDisplay=10000  ReferenceConstellation="{[0.70711+0.70711i        -0.70711+0.70711i        -0.70711-0.70711i         0.70711-0.70711i],[0.70711+0.70711i        -0.70711+0.70711i        -0.70711-0.70711i         0.70711-0.70711i]}"  ReferenceMarker={''+'',''+''}  ReferenceColor={[1 0 0],[1 0 0]}  XLimits=[-1.3581 1.3569]  YLimits=[-1.3581 1.3569]  AxesLimits=[-1.3581 1.3569]  ShowLegend=on  DefaultConfigurationName=comm.scopes.ConstellationDiagramBlockCfg
      settings: OpenAtSimulationStart=off
  Subsystem : Subsystem
  Unit Delay Enabled Synchronous : hdlsllib/Discrete/Unit Delay Enabled Synchronous  InitialCondition=0.0  SampleTime=-1
  Unit Delay Enabled Synchronous1 : hdlsllib/Discrete/Unit Delay Enabled Synchronous  InitialCondition=0.0  SampleTime=-1
  wires:
  In4/1 -> Unit Delay Enabled Synchronous1/2, Subsystem/Enable
  Data Type Conversion/1 -> Unit Delay Enabled Synchronous1/1, Subsystem/1(In1)
  Unit Delay Enabled Synchronous1/1 -> QPSK Receiver Constellations 2/2  "After Carrier Synchronization"
  In2/1 -> Unit Delay Enabled Synchronous/2
  In1/1 -> Data Type Conversion1/1
  Data Type Conversion1/1 -> Unit Delay Enabled Synchronous/1
  Unit Delay Enabled Synchronous/1 -> QPSK Receiver Constellations 2/1  "After Symbol Synchronization"
  In3/1 -> Data Type Conversion/1

== system sim_internal_baseline_TB/Receiver/QPSK Rx/Frequency and Time Synchronizer/Packet Controller ==
  dataIn : Inport
  syncPulse : Inport  Port=2
  validIn : Inport  Port=3
  Delay : Delay  DelayLength=4
  Delay1 : Delay  DelayLength=4
  Delay2 : Delay  DelayLength=4
  End Generator : Subsystem
  Logical Operator : Logic  IconShape=distinctive  AllPortsSameDT=off  OutDataTypeStr=boolean
  MATLAB Function : MATLAB Function  TreatAsAtomicUnit=on
  Time Scope End Generator : Scope  Commented=on  NumInputPorts=2
      settings: SampleTime=1  ActiveDisplayYMinimum=-0.048155737704917989  ActiveDisplayYMaximum=1.0464480874316939  YLabel=Amplitude  DataLoggingVariableName=ScopeData2
  To File : ToFile  Filename=end_gen.mat  MatrixName=end_gen  SaveFormat=Timeseries
  To File1 : ToFile  Filename=reset  MatrixName=reset  SaveFormat=Timeseries
  sample discard controller : MATLAB Function  TreatAsAtomicUnit=on
  dataOut : Outport
  startOut : Outport  Port=2
  endOut : Outport  Port=3
  validOut : Outport  Port=4
  wires:
  MATLAB Function/1(out) -> Logical Operator/2
  sample discard controller/1(dataOut) -> dataOut/1
  sample discard controller/2(startOut) -> startOut/1
  sample discard controller/3(endOut) -> endOut/1
  sample discard controller/4(validOut) -> validOut/1
  Delay/1 -> sample discard controller/1(dataIn)
  Delay1/1 -> sample discard controller/2(validIn), End Generator/1(validIn)
  Delay2/1 -> sample discard controller/3(startIn)
  dataIn/1 -> Delay/1
  validIn/1 -> MATLAB Function/1(valid), Delay1/1, Logical Operator/1
  Logical Operator/1 -> Delay2/1, To File1/1, Time Scope End Generator/2, End Generator/2(rst)
  syncPulse/1 -> MATLAB Function/2(syncPulse)
  End Generator/1(endOut) -> Time Scope End Generator/1, To File/1, sample discard controller/4(endIn)

== system sim_internal_baseline_TB/Receiver/QPSK Rx/Frequency and Time Synchronizer/Phase Ambiguity Estimation and Correction ==
  dataIn : Inport
  syncPulseIn : Inport  Port=2
  validIn : Inport  Port=3
  Average Estimates : Subsystem
  Delay : Delay  DelayLength=32
  Delay1 : Delay  DelayLength=32
  Delay10 : Delay  DelayLength=15 + 7
  Delay11 : Delay  DelayLength=5
  Delay12 : Delay  DelayLength=5
  Delay13 : Delay  DelayLength=5
  Delay2 : Delay  DelayLength=32
  Delay3 : Delay  DelayLength=8
  Delay4 : Delay  DelayLength=8
  Delay5 : Delay  DelayLength=8
  Delay6 : Delay  DelayLength=1
  Delay7 : Delay  DelayLength=1
  Delay8 : Delay  DelayLength=1
  Delay9 : Delay  DelayLength=10
  Phase Ambiguity Corrector : Subsystem
  Phase Ambiguity Estimator : Subsystem
  dataOut : Outport
  syncPulseOut : Outport  Port=2
  validOut : Outport  Port=3
  wires:
  Delay4/1 -> Delay2/1
  Delay5/1 -> Delay/1
  Delay3/1 -> Delay1/1
  Delay10/1 -> Delay9/1
  Phase Ambiguity Corrector/1(dataOut) -> dataOut/1
  Phase Ambiguity Corrector/2(validOut) -> validOut/1
  Delay9/1 -> syncPulseOut/1
  Delay8/1 -> Phase Ambiguity Corrector/1(dataIn)
  Average Estimates/1(avgEst) -> Phase Ambiguity Corrector/2(estimate)
  Delay7/1 -> Phase Ambiguity Corrector/3(validIn)
  Delay6/1 -> Delay10/1
  dataIn/1 -> Delay5/1
  validIn/1 -> Delay4/1
  Delay13/1 -> Delay8/1
  Phase Ambiguity Estimator/1(endOut) -> Average Estimates/1(endIn)
  Phase Ambiguity Estimator/3(validOut) -> Average Estimates/3(validIn)
  Delay12/1 -> Delay7/1
  Delay11/1 -> Delay6/1
  Phase Ambiguity Estimator/2(estOut) -> Average Estimates/2(estin)
  Delay/1 -> Delay13/1, Phase Ambiguity Estimator/1(dataIn)
  syncPulseIn/1 -> Phase Ambiguity Estimator/2(syncPulse), Delay3/1
  Delay2/1 -> Phase Ambiguity Estimator/3(validIn), Delay12/1
  Delay1/1 -> Delay11/1

== system sim_internal_baseline_TB/Receiver/QPSK Rx/Frequency and Time Synchronizer/Preamble Detector ==
  dataIn : Inport
  validIn : Inport  Port=2
  Constant : Constant  Value=false  SampleTime=-1
  Correlator : Subsystem
  Delay : Delay  DelayLength=20
  Delay{1..5,11..14} (9 alike) : Delay  DelayLength=1
  Delay10 : Delay  DelayLength=searchSamples * 4
  Delay6 : Delay  DelayLength=6
  Delay7 : Delay  DelayLength=20
  Delay8 : Delay  DelayLength=6
  FIFO : Subsystem  mask{fifoSize=searchSamples, pushFullDiag=Error, popEmptyDiag=Error}
      mask prompts: fifoSize "FIFO size:"; pushFullDiag "Push full FIFO:"; popEmptyDiag "Pop empty FIFO:"
      mask TypeOptions pushFullDiag: Ignore | Warning | Error
      mask TypeOptions popEmptyDiag: Ignore | Warning | Error
  Logical Operator : Logic  AllPortsSameDT=off  OutDataTypeStr=boolean
  No HDL : Subsystem
  Peak Search : Subsystem  VariantControl=new  mask{samplesPerFrame=searchSamples}
      mask prompts: samplesPerFrame "Number of samples to search:"
      mask init:
      | samplesPerFrame1x            = samplesPerFrame;
      |     searchDuration               = samplesPerFrame1x;
  Relational Operator : RelationalOperator  Operator=>  OutDataTypeStr=boolean  InputSameDT=off
  Terminator : Terminator
  Terminator1 : Terminator
  Timing Adjust : Subsystem
  dataOut : Outport
  syncPulse : Outport  Port=2
  validOut : Outport  Port=3
  wires:
  Delay/1 -> Delay6/1
  validIn/1 -> Delay2/1
  dataIn/1 -> Delay1/1
  Relational Operator/1 -> Peak Search/2(thresholdExceeded)
  Peak Search/3(success) -> Logical Operator/2  "success"
  Peak Search/2(done) -> Logical Operator/1  "done"
  Delay7/1 -> Delay8/1
  Timing Adjust/1(dataOut) -> Delay3/1  "synchronizedData"
  Timing Adjust/3(SyncPulse) -> Delay4/1  "synchronizedPulse"
  Timing Adjust/2(validOut) -> Delay5/1  "synchronizedValid"
  Delay3/1 -> dataOut/1
  Delay5/1 -> validOut/1
  Delay4/1 -> syncPulse/1
  Peak Search/1(timingOffset) -> Delay11/1
  Logical Operator/1 -> Delay12/1
  Delay10/1 -> FIFO/3(pop), Delay14/1
  Correlator/3(validOut) -> Peak Search/3(validIn), No HDL/Enable
  Correlator/2(threshold) -> Relational Operator/2, No HDL/2(In2)
  Correlator/1(dataOut) -> Relational Operator/1, Peak Search/1(corr), No HDL/1(In1)
  Delay8/1 -> FIFO/2(push), Delay10/1
  Delay1/1 -> Delay/1, Correlator/1(dataIn)
  Delay2/1 -> Delay7/1, Correlator/2(validIn)
  Delay11/1 -> Timing Adjust/1(timingOffset)
  Delay12/1 -> Timing Adjust/2(timingOffsetValid)
  Delay13/1 -> Timing Adjust/3(dataIn)
  Delay14/1 -> Timing Adjust/4(validIn)
  FIFO/2(numEntries) -> Terminator/1
  Constant/1 -> FIFO/4(reset)
  FIFO/3(validPop) -> Terminator1/1
  Delay6/1 -> FIFO/1(in)
  FIFO/1(out) -> Delay13/1

== system sim_internal_baseline_TB/Receiver/QPSK Rx/Frequency and Time Synchronizer/Symbol Synchronizer ==
  dataIn : Inport
  validIn : Inport  Port=2
  Data Type Conversion4 : DataTypeConversion  OutDataTypeStr=fixdt(1,16,14)  SaturateOnIntegerOverflow=off  RndMeth=Floor
  Delay{1..4,6,8..9} (7 alike) : Delay  DelayLength=1
  Delay5 : Delay  DelayLength=12
  Delay7 : Delay  DelayLength=12
  Gardner TED : Subsystem
  Integer Delay{1..4} (4 alike) : Delay  DelayLength=1
  Interpolation Control : MATLAB Function
  Interpolation Filter : Subsystem
  Loop Filter : Subsystem
  No HDL : Subsystem
  Rate Handle : Subsystem
  dataOut : Outport
  validOut : Outport  Port=2
  wires:
  Loop Filter/1(v) -> Delay4/1
  Gardner TED/1(e) -> Delay3/1
  Interpolation Control/2(Underflow) -> Integer Delay3/1
  Integer Delay4/1 -> Interpolation Filter/2(mu)
  dataIn/1 -> No HDL/1(data), Integer Delay1/1
  Integer Delay3/1 -> Delay5/1
  Delay3/1 -> Loop Filter/1(e)
  Delay4/1 -> Interpolation Control/1(Delta)
  Data Type Conversion4/1 -> Rate Handle/1(dataIn)
  Delay1/1 -> Data Type Conversion4/1
  Delay6/1 -> Rate Handle/3(validIn)
  Delay7/1 -> Delay6/1
  validIn/1 -> No HDL/2(valid), Integer Delay2/1
  Rate Handle/2(validOut) -> validOut/1
  Rate Handle/1(dataOut) -> dataOut/1
  Interpolation Filter/1(interpolant) -> Delay8/1, Delay1/1
  Interpolation Control/1(mu) -> Integer Delay4/1
  Delay2/1 -> Rate Handle/2(strobe)
  Delay5/1 -> Delay9/1, Delay2/1
  Integer Delay1/1 -> Interpolation Filter/1(In)
  Integer Delay2/1 -> Delay7/1
  Delay8/1 -> Gardner TED/1(data)
  Delay9/1 -> Gardner TED/2(strobe)

== system sim_internal_baseline_TB/Receiver/QPSK Rx/QPSK Demodulator/Serializer ==
  u : Inport
  In2 : Inport  Port=2
  Delay1 : Delay  DelayLength=1
  Delay4 : Delay  DelayLength=1
  Demux : Demux  Outputs=2
  HDL Counter : hdlsllib/Sources/HDL Counter  CountType=Count limited  CountInit=0  CountStep=1  CountMax=1  CountFromType=Initial value  CountFrom=0  CountResetPort=off  CountLoadPort=off  CountEnbPort=on  CountDirPort=off  CountHitOutputPort=off  CountDataType=Unsigned  CountWordLen=1  CountFracLen=0  CountSampTime=1
  Logical Operator : Logic  Operator=OR  AllPortsSameDT=off  OutDataTypeStr=boolean
  Multiport Switch : MultiPortSwitch  DataPortOrder=Zero-based contiguous  Inputs=2  zeroidx=on  SaturateOnIntegerOverflow=off  InputSameDT=off
  Unit Delay Enabled Synchronous : hdlsllib/Discrete/Unit Delay Enabled Synchronous  InitialCondition=0.0  SampleTime=-1
  Out1 : Outport
  Out2 : Outport  Port=2
  wires:
  Demux/2 -> Multiport Switch/3
  Logical Operator/1 -> Out2/1, HDL Counter/1
  In2/1 -> Unit Delay Enabled Synchronous/2, Delay1/1
  HDL Counter/1 -> Multiport Switch/1
  Delay4/1 -> Logical Operator/2
  u/1 -> Unit Delay Enabled Synchronous/1
  Multiport Switch/1 -> Out1/1
  Demux/1 -> Multiport Switch/2
  Delay1/1 -> Logical Operator/1, Delay4/1
  Unit Delay Enabled Synchronous/1 -> Demux/1
